simulink model "DISCRRETE_PID"  (R2024b)
settings: Solver=VariableStepAuto  StartTime=0.0  StopTime=15  RelTol=1e-3
undefined symbols (not defined in the file): b, J, Kd, ke, Ki, Kp, kt, L, Nf, R
settings Model: Creator=omari  LastModifiedBy=omari

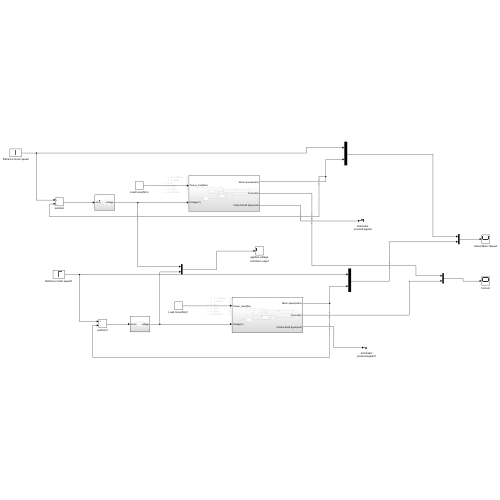
[thumbnail: Simulink's stored preview of the top-level diagram]
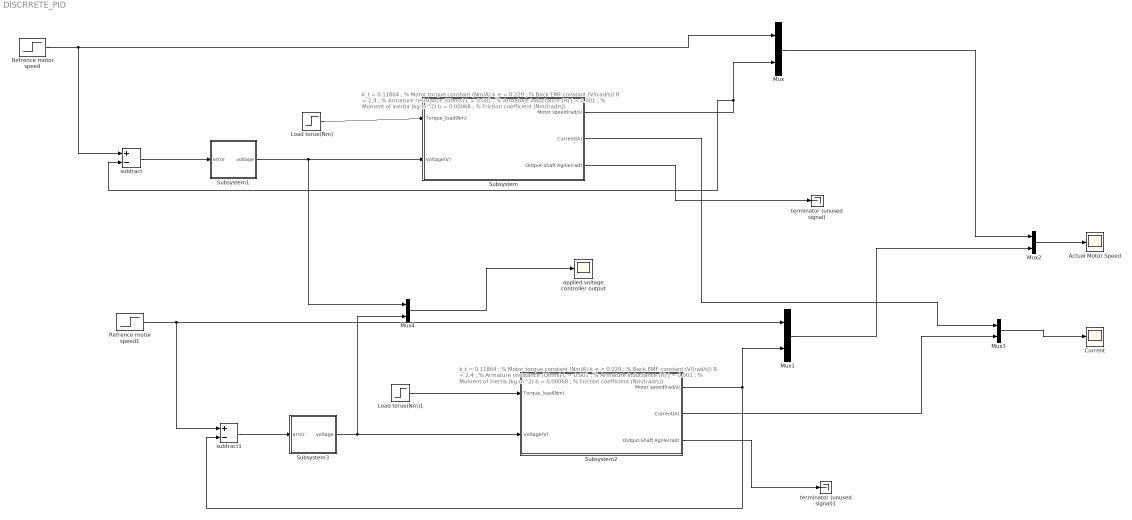
== system DISCRRETE_PID ==
  note: k_t = 0.11864 ; % Motor torque constant (Nm/A)
      | k_e = 0.229 ; % Back EMF constant (V/(rad/s))
      | R = 2.4 ; % Armature resistance (Ohms)
      | L = 0.001 ; % Armature inductance (H)
      | J = 0.001 ; % Moment of inertia (kg.m^2)
      | b = 0.00068 ; % Friction coefficient (Nm/(rad/s))
  note: k_t = 0.11864 ; % Motor torque constant (Nm/A)
      | k_e = 0.229 ; % Back EMF constant (V/(rad/s))
      | R = 2.4 ; % Armature resistance (Ohms)
      | L = 0.001 ; % Armature inductance (H)
      | J = 0.001 ; % Moment of inertia (kg.m^2)
      | b = 0.00068 ; % Friction coefficient (Nm/(rad/s))
  Actual Motor Speed : Scope
  Current : Scope
  Load torue(Nm) : Step  Time=15  After=0.25  SampleTime=0
  Load torue(Nm)1 : Step  Time=15  After=0.25  SampleTime=0
  Mux{,1..4} (5 alike) : Mux  Inputs=2
  Refrence motor speed : Step  After=31.42  SampleTime=0.5
  Refrence motor speed1 : Step  After=31.42  SampleTime=0.5
  Subsystem : Subsystem
  Subsystem1 : Subsystem
  Subsystem2 : Subsystem
  Subsystem3 : Subsystem
  applied voltage controller output : Scope
  subtract : Sum  Inputs=+-
  subtract1 : Sum  Inputs=+-
  terminator (unused signal) : Terminator
  terminator (unused signal)1 : Terminator
  wires:
  Subsystem/3(OUtput-Shaft Agnle(rad)) -> terminator (unused signal)/1
  Subsystem/1(Motor speed(rad/s)) -> Mux/2, subtract/2
  subtract/1 -> Subsystem1/1(error)
  Subsystem1/1(voltage) -> Mux4/1, Subsystem/2(Voltage(V))
  Load torue(Nm)/1 -> Subsystem/1(Torque_load(Nm))
  Refrence motor speed/1 -> subtract/1, Mux/1
  Refrence motor speed1/1 -> subtract1/1, Mux1/1
  subtract1/1 -> Subsystem3/1(error)
  Subsystem3/1(voltage) -> Subsystem2/2(Voltage(V)), Mux4/2
  Subsystem2/1(Motor speed(rad/s)) -> Mux1/2, subtract1/2
  Subsystem2/3(OUtput-Shaft Agnle(rad)) -> terminator (unused signal)1/1
  Load torue(Nm)1/1 -> Subsystem2/1(Torque_load(Nm))
  Mux/1 -> Mux2/1
  Mux1/1 -> Mux2/2
  Mux2/1 -> Actual Motor Speed/1
  Subsystem/2(Current(A)) -> Mux3/1
  Subsystem2/2(Current(A)) -> Mux3/2
  Mux3/1 -> Current/1
  Mux4/1 -> applied voltage controller output/1

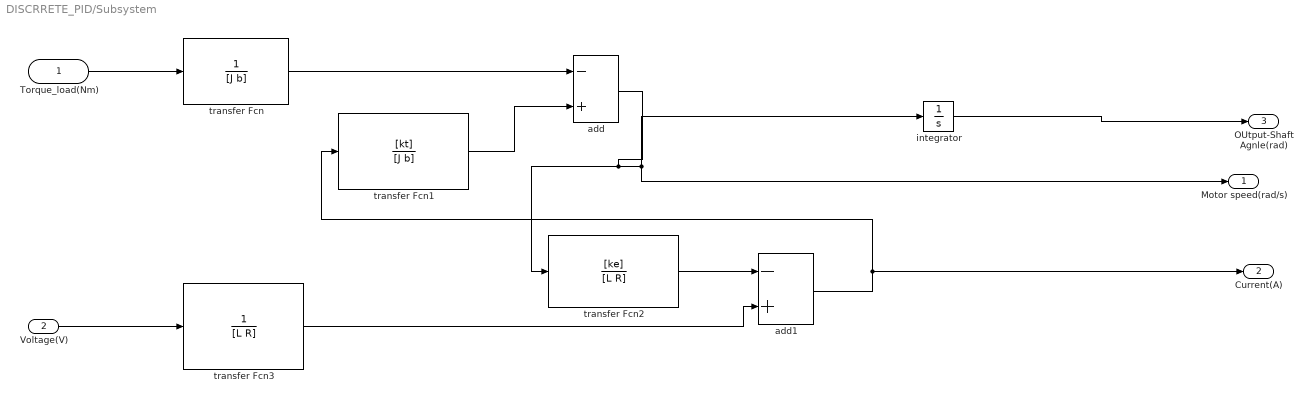
== system DISCRRETE_PID/Subsystem ==
  Torque_load(Nm) : Inport
  Voltage(V) : Inport  Port=2
  add : Sum  Inputs=-+
  add1 : Sum  Inputs=-+
  integrator : Integrator
  transfer Fcn : TransferFcn  Denominator=[J b]
  transfer Fcn1 : TransferFcn  Numerator=[kt]  Denominator=[J b]
  transfer Fcn2 : TransferFcn  Numerator=[ke]  Denominator=[L R]
  transfer Fcn3 : TransferFcn  Denominator=[L R]
  Motor speed(rad/s) : Outport
  Current(A) : Outport  Port=2
  OUtput-Shaft Agnle(rad) : Outport  Port=3
  wires:
  add/1 -> transfer Fcn2/1, Motor speed(rad/s)/1, integrator/1
  add1/1 -> Current(A)/1, transfer Fcn1/1
  Torque_load(Nm)/1 -> transfer Fcn/1
  transfer Fcn3/1 -> add1/2
  transfer Fcn2/1 -> add1/1
  Voltage(V)/1 -> transfer Fcn3/1
  transfer Fcn/1 -> add/1
  transfer Fcn1/1 -> add/2
  integrator/1 -> OUtput-Shaft Agnle(rad)/1

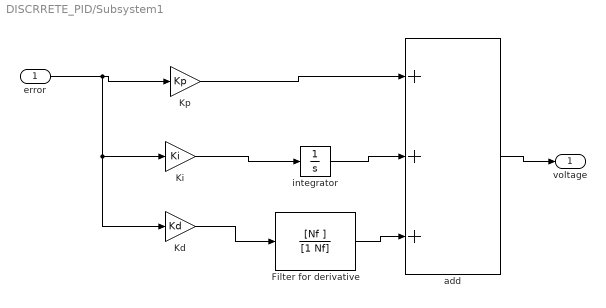
== system DISCRRETE_PID/Subsystem1 ==
  error : Inport
  Filter for derivative : TransferFcn  Numerator=[Nf ]  Denominator=[1 Nf]
  Kd : Gain  Gain=Kd
  Ki : Gain  Gain=Ki
  Kp : Gain  Gain=Kp
  add : Sum  Inputs=+++
  integrator : Integrator
  voltage : Outport
  wires:
  error/1 -> Kd/1, Ki/1, Kp/1
  Filter for derivative/1 -> add/3
  Kd/1 -> Filter for derivative/1
  Kp/1 -> add/1
  integrator/1 -> add/2
  Ki/1 -> integrator/1
  add/1 -> voltage/1

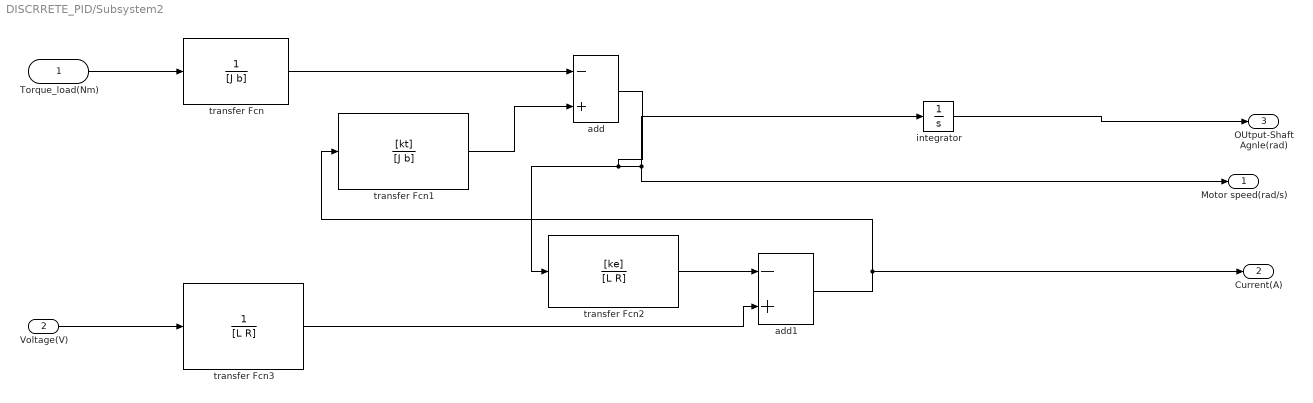
== system DISCRRETE_PID/Subsystem2 ==
  Torque_load(Nm) : Inport
  Voltage(V) : Inport  Port=2
  add : Sum  Inputs=-+
  add1 : Sum  Inputs=-+
  integrator : Integrator
  transfer Fcn : TransferFcn  Denominator=[J b]
  transfer Fcn1 : TransferFcn  Numerator=[kt]  Denominator=[J b]
  transfer Fcn2 : TransferFcn  Numerator=[ke]  Denominator=[L R]
  transfer Fcn3 : TransferFcn  Denominator=[L R]
  Motor speed(rad/s) : Outport
  Current(A) : Outport  Port=2
  OUtput-Shaft Agnle(rad) : Outport  Port=3
  wires:
  add/1 -> transfer Fcn2/1, Motor speed(rad/s)/1, integrator/1
  add1/1 -> Current(A)/1, transfer Fcn1/1
  Torque_load(Nm)/1 -> transfer Fcn/1
  transfer Fcn3/1 -> add1/2
  transfer Fcn2/1 -> add1/1
  Voltage(V)/1 -> transfer Fcn3/1
  transfer Fcn/1 -> add/1
  transfer Fcn1/1 -> add/2
  integrator/1 -> OUtput-Shaft Agnle(rad)/1

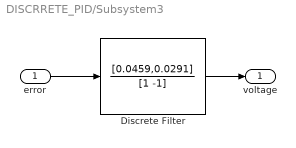
== system DISCRRETE_PID/Subsystem3 ==
  error : Inport
  Discrete Filter : DiscreteFilter  Numerator=[0.0459,0.0291]  Denominator=[1 -1]
  voltage : Outport
  wires:
  Discrete Filter/1 -> voltage/1
  error/1 -> Discrete Filter/1
